simulink model "Integrated_Joystick_SIM"  (R2025b)
settings: Solver=FixedStepDiscrete  StartTime=0.0  StopTime=tspan  FixedStep=dt_sim  RelTol=1e-3
undefined symbols (not defined in the file): const_voltage, mission_file
settings Model: Creator=vulcangrip  LastModifiedBy=vulcangrip
settings OptimizationCC: DefaultParameterBehavior=Inlined  EnhancedBackFolding=on  PassReuseOutputArgsAs=Individual arguments  ZeroExternalMemoryAtStartup=off  ZeroInternalMemoryAtStartup=off  MaxStackSize=64  OptimizeBlockOrder=speed  DifferentSizesBufferReuse=on  OptimizationCustomize=off  EfficientTunableParamExpr=on
settings DebuggingCC: ParameterTunabilityLossMsg=error
settings HardwareCC: ProdBitPerLong=64.0  ProdHWDeviceType=Intel->x86-64 (Linux 64)
settings SFSimCC: MATLABDynamicMemAlloc=off  SimTargetLang=C++  SimDLTargetLibrary=mkl-dnn
settings RTWCC: SystemTargetFile=ert.tlc  HardwareBoard=Robot Operating System 2 (ROS 2)  TLCOptions="-aInlineSetEventsForThisBaseRateFcn=TLC_FALSE -aSuppressMultiTaskScheduler=TLC_FALSE  -aRateBasedStepFcn=0"  GenCodeOnly=on  TemplateMakefile=ert_default_tmf  Toolchain=Colcon Tools  TargetLang=C++  CheckMdlBeforeBuild=Warning  Description=Embedded Coder
settings CodeAppCC: ForceParamTrailComments=on  IgnoreCustomStorageClasses=off  OperatorAnnotations=on  SimulinkDataObjDesc=on  SFDataObjDesc=on  InsertBlockDesc=on
settings ERTTargetCC: ExtModeTransport=2.0  ExtModeStaticAlloc=on  ExtModeAutomaticAllocSize=off  ExtModeMexFile=ext_xcp  ExtModeIntrfLevel=Level2 - Open  RootIOFormat=Structure reference  TargetLangStandard=C++11 (ISO)  CodeInterfacePackaging=C++ class  SubcomponentCodeInterfacePackaging=C++ class

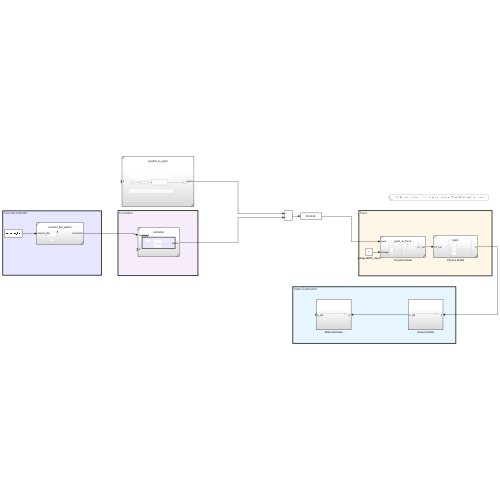
[thumbnail: Simulink's stored preview of the top-level diagram]
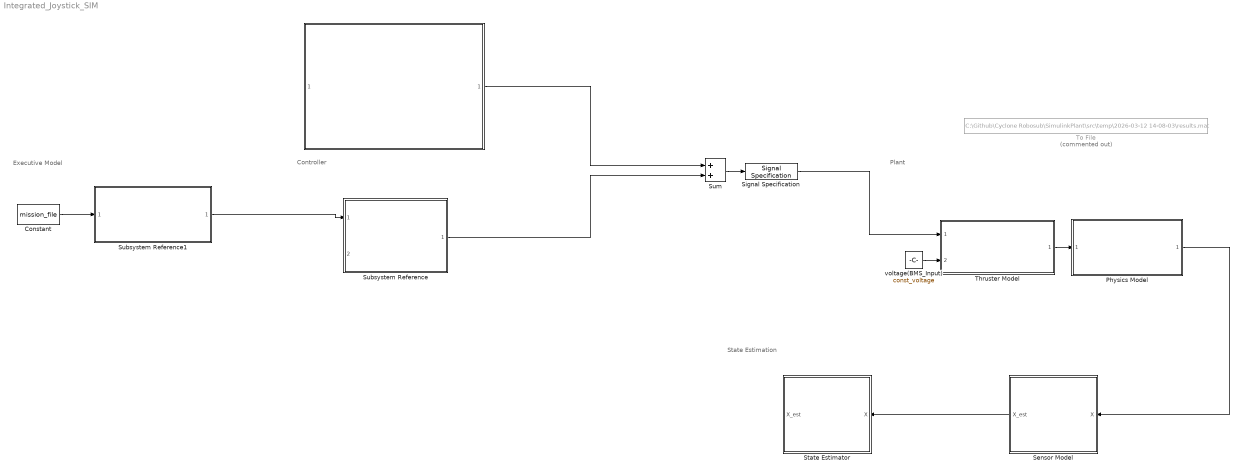
== system Integrated_Joystick_SIM ==
  note: Controller
  note: Executive Model
  note: State Estimation
  note: Plant
  " " : Subsystem  ReferencedSubsystem=joystick_to_pwm
  Constant : Constant  Value=mission_file
  Physics Model : Subsystem  ReferencedSubsystem=plant
  Sensor Model : Subsystem
  Signal Specification : SignalSpecification  OutDataTypeStr=int32
  State Estimator : Subsystem
  Subsystem Reference : Subsystem  ReferencedSubsystem=controller
  Subsystem Reference1 : Subsystem  ReferencedSubsystem=mission_file_parser
  Sum : Sum
  Thruster Model : Subsystem  ReferencedSubsystem=pwm_to_force
  To File : ToFile  Commented=on  Filename=C:\Github\Cyclone Robosub\SimulinkPlant\src\temp\2026-03-12 14-08-03\results.mat  MatrixName=X  SaveFormat=Timeseries
  voltage(BMS_Input) : Constant  Value=const_voltage
  wires:
  Sensor Model/1(X_est) -> State Estimator/1(X)
  Constant/1 -> Subsystem Reference1/1
  Physics Model/1 -> Sensor Model/1(X)
  Thruster Model/1 -> Physics Model/1
  Subsystem Reference1/1 -> Subsystem Reference/1
  voltage(BMS_Input)/1 -> Thruster Model/2
  Sum/1 -> Signal Specification/1
  " "/1 -> Sum/1
  Subsystem Reference/1 -> Sum/2
  Signal Specification/1 -> Thruster Model/1

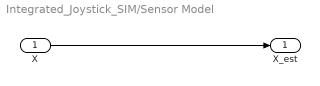
== system Integrated_Joystick_SIM/Sensor Model ==
  X : Inport
  X_est : Outport
  wires:
  X/1 -> X_est/1

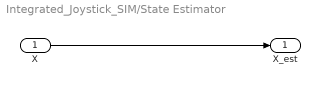
== system Integrated_Joystick_SIM/State Estimator ==
  X : Inport
  X_est : Outport
  wires:
  X/1 -> X_est/1
